simulink library "csc_hmg_homoraphy_meas_lib"  (R2015b)
settings: Solver=ode45  SolverMode=SingleTasking  StartTime=0.0  StopTime=10.0  RelTol=1e-3
values from neighbouring files (symbols this model uses):
  fsp_camera_alt_cutoff = 5    [csc_snp_sensor_prep_init.m]
  hmg_img1_delay_cnts = round(0.1 / est_time_step)    [csc_snp_sensor_prep_init.m]
  snp_fsp_index = [ 2 3 ]    [csc_snp_sensor_prep_init.m]
  snp_fsp_zero_index = [ 0 0 ]    [csc_snp_sensor_prep_init.m]
undefined symbols (not defined in the file or in its folder): cam_cam1_lander_dcm, cam_image_plane_norm, kfl_use_camera_meas
libraries: simulink x2, util_info_lib x2, csu_htv_homography_to_velocity_lib x2, csu_und_unduplicate_lib x2, util_common_lib x2
settings Model: ExtModeAutoUpdateStatusClock=off  Creator=Administrator  LastModifiedBy=Mark Agbayani
settings DataIOCC: SaveFormat=Array  SignalLoggingSaveFormat=ModelDataLogs
settings OptimizationCC: BlockReduction=off  BooleanDataType=off  ExpressionDepthLimit=2147483647
settings DebuggingCC: SaveWithParameterizedLinksMsg=none  UnderspecifiedInitializationDetection=Classic  MergeDetectMultiDrivingBlocksExec=none  SignalResolutionControl=TryResolveAllWithWarning  FcnCallInpInsideContextMsg=EnableAllAsWarning  StateNameClashWarn=warning  StrictBusMsg=Warning
settings HardwareCC: ProdBitPerPointer=32  ProdLargestAtomicFloat=None  ProdIntDivRoundTo=Undefined  ProdEndianess=Unspecified  ProdWordSize=32  ProdHWDeviceType=32-bit Generic  TargetUnknown=on
settings GRTTargetCC: GeneratePreprocessorConditionals=Disable all  CombineOutputUpdateFcns=off  GRTInterface=on
settings ConfigComp: CovModelRefEnable=Off  CovSFcnEnable=off

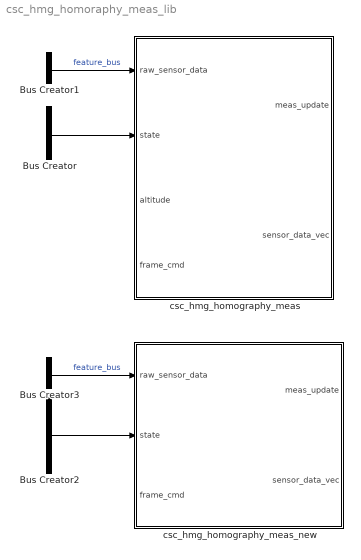
== system csc_hmg_homoraphy_meas_lib ==
  Bus Creator : BusCreator  Inputs=4
  Bus Creator1 : BusCreator  Inputs=2  OutDataTypeStr=Bus: feature_msg  NonVirtualBus=on
  Bus Creator2 : BusCreator  Inputs=5
  Bus Creator3 : BusCreator  Inputs=2  OutDataTypeStr=Bus: feature_msg  NonVirtualBus=on
  csc_hmg_homography_meas : Subsystem
  csc_hmg_homography_meas_new : Subsystem
  wires:
  ? -> Bus Creator/2  "accel"
  ? -> Bus Creator/3  "rate"
  ? -> Bus Creator/1  "x"
  ? -> Bus Creator/4  "q"
  Bus Creator/1 -> csc_hmg_homography_meas/2(state)
  ? -> Bus Creator1/2  "pixels_2"
  ? -> Bus Creator1/1  "pixels_1"
  Bus Creator1/1 -> csc_hmg_homography_meas/1(raw_sensor_data)  "feature_bus"
  ? -> Bus Creator2/2  "accel"
  ? -> Bus Creator2/3  "rate"
  ? -> Bus Creator2/1  "x"
  ? -> Bus Creator2/4  "q"
  Bus Creator2/1 -> csc_hmg_homography_meas_new/2(state)
  ? -> Bus Creator3/2  "pixels_2"
  ? -> Bus Creator3/1  "pixels_1"
  Bus Creator3/1 -> csc_hmg_homography_meas_new/1(raw_sensor_data)  "feature_bus"
  ? -> Bus Creator2/5  "altitude"

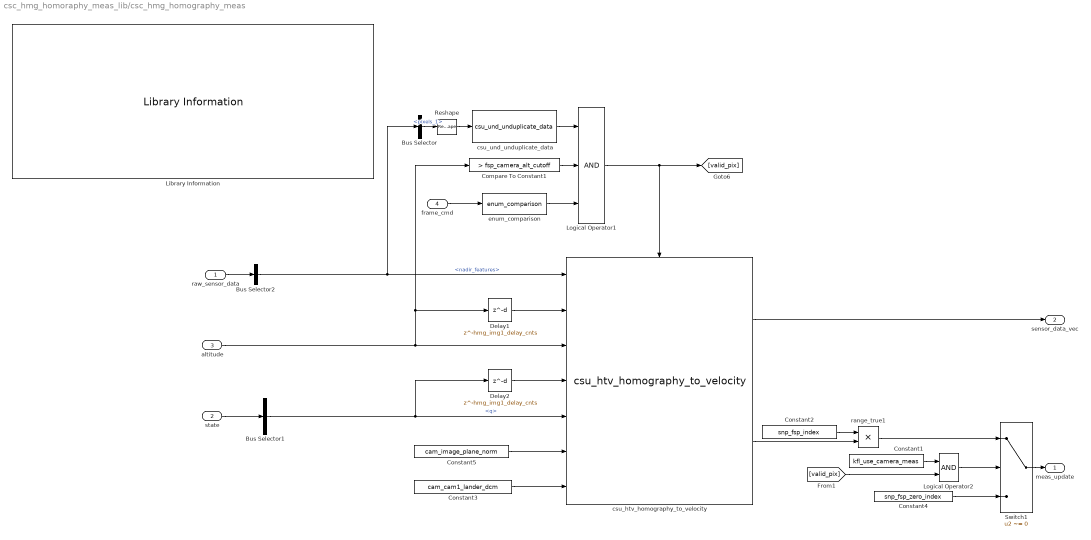
== system csc_hmg_homoraphy_meas_lib/csc_hmg_homography_meas ==
  raw_sensor_data : Inport
  state : Inport  Port=2
  altitude : Inport  Port=3
  frame_cmd : Inport  Port=4
  Bus Selector : BusSelector  OutputSignals=pixels_1
  Bus Selector1 : BusSelector  OutputSignals=q
  Bus Selector2 : BusSelector  OutputSignals=nadir_features
  Compare To Constant1 : simulink/Logic and Bit Operations/Compare To Constant  relop=>  const=fsp_camera_alt_cutoff  OutDataTypeStr=uint8
  Constant1 : Constant  Value=kfl_use_camera_meas
  Constant2 : Constant  Value=snp_fsp_index
  Constant3 : Constant  Value=cam_cam1_lander_dcm
  Constant4 : Constant  Value=snp_fsp_zero_index
  Constant5 : Constant  Value=cam_image_plane_norm  VectorParams1D=off
  Delay1 : Delay  DelayLength=hmg_img1_delay_cnts
  Delay2 : Delay  DelayLength=hmg_img1_delay_cnts
  Library Information : util_info_lib/Library Information  owner='NONE'
  Logical Operator1 : Logic  Inputs=3  AllPortsSameDT=off  OutDataTypeStr=boolean
  Logical Operator2 : Logic  AllPortsSameDT=off  OutDataTypeStr=boolean
  Reshape : Reshape
  Switch1 : Switch  Criteria=u2 ~= 0
  csu_htv_homography_to_velocity : csu_htv_homography_to_velocity_lib/csu_htv_homography_to_velocity
  csu_und_unduplicate_data : csu_und_unduplicate_lib/csu_und_unduplicate_data  initial_compare=0
  enum_comparison : util_common_lib/enum_comparison  comparison_type===
  range_true1 : Product  RndMeth=Zero
  meas_update : Outport
  sensor_data_vec : Outport  Port=2
  wires:
  [valid_pix] -> Logical Operator2/2
  Logical Operator2/1 -> Switch1/2
  Constant1/1 -> Logical Operator2/1
  Constant2/1 -> range_true1/1
  range_true1/1 -> Switch1/1
  csu_htv_homography_to_velocity/2 -> range_true1/2
  Delay2/1 -> csu_htv_homography_to_velocity/4
  frame_cmd/1 -> enum_comparison/1
  enum_comparison/1 -> Logical Operator1/3
  Constant3/1 -> csu_htv_homography_to_velocity/7
  Bus Selector2/1 -> csu_htv_homography_to_velocity/1, Bus Selector/1  "<nadir_features>"
  raw_sensor_data/1 -> Bus Selector2/1
  Constant5/1 -> csu_htv_homography_to_velocity/6
  Delay1/1 -> csu_htv_homography_to_velocity/2
  Bus Selector/1 -> Reshape/1  "<pixels_1>"
  Switch1/1 -> meas_update/1
  csu_htv_homography_to_velocity/1 -> sensor_data_vec/1
  Constant4/1 -> Switch1/3
  Compare To Constant1/1 -> Logical Operator1/2
  csu_und_unduplicate_data/1 -> Logical Operator1/1
  Logical Operator1/1 -> [valid_pix], csu_htv_homography_to_velocity/Enable
  Reshape/1 -> csu_und_unduplicate_data/1
  state/1 -> Bus Selector1/1
  Bus Selector1/1 -> csu_htv_homography_to_velocity/5, Delay2/1  "<q>"
  altitude/1 -> csu_htv_homography_to_velocity/3, Delay1/1, Compare To Constant1/1

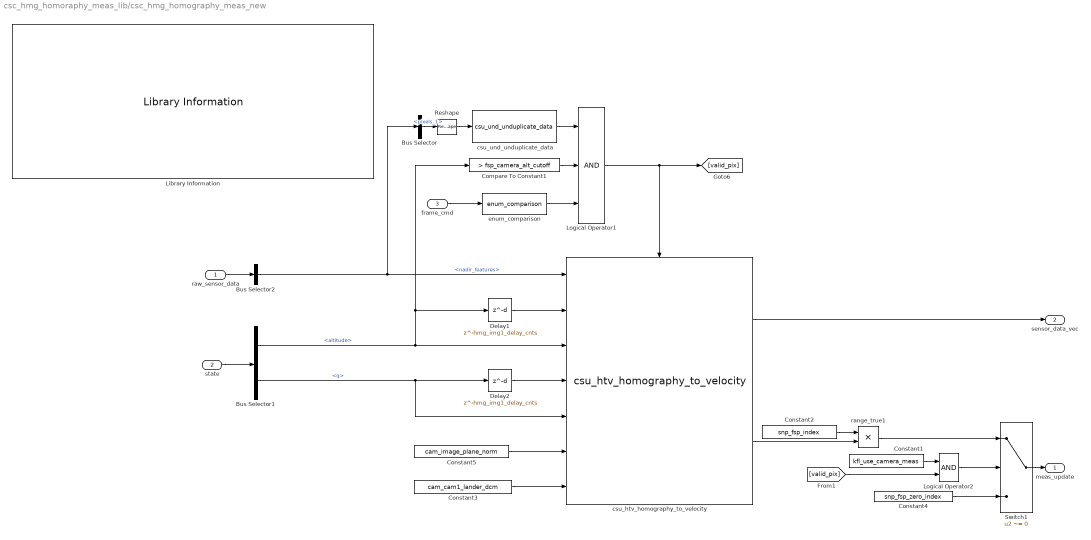
== system csc_hmg_homoraphy_meas_lib/csc_hmg_homography_meas_new ==
  raw_sensor_data : Inport
  state : Inport  Port=2
  frame_cmd : Inport  Port=3
  Bus Selector : BusSelector  OutputSignals=pixels_1
  Bus Selector1 : BusSelector  OutputSignals=altitude,q
  Bus Selector2 : BusSelector  OutputSignals=nadir_features
  Compare To Constant1 : simulink/Logic and Bit Operations/Compare To Constant  relop=>  const=fsp_camera_alt_cutoff  OutDataTypeStr=uint8
  Constant1 : Constant  Value=kfl_use_camera_meas
  Constant2 : Constant  Value=snp_fsp_index
  Constant3 : Constant  Value=cam_cam1_lander_dcm
  Constant4 : Constant  Value=snp_fsp_zero_index
  Constant5 : Constant  Value=cam_image_plane_norm  VectorParams1D=off
  Delay1 : Delay  DelayLength=hmg_img1_delay_cnts
  Delay2 : Delay  DelayLength=hmg_img1_delay_cnts
  Library Information : util_info_lib/Library Information  owner='NONE'
  Logical Operator1 : Logic  Inputs=3  AllPortsSameDT=off  OutDataTypeStr=boolean
  Logical Operator2 : Logic  AllPortsSameDT=off  OutDataTypeStr=boolean
  Reshape : Reshape
  Switch1 : Switch  Criteria=u2 ~= 0
  csu_htv_homography_to_velocity : csu_htv_homography_to_velocity_lib/csu_htv_homography_to_velocity
  csu_und_unduplicate_data : csu_und_unduplicate_lib/csu_und_unduplicate_data  initial_compare=0
  enum_comparison : util_common_lib/enum_comparison  comparison_type===
  range_true1 : Product  RndMeth=Zero
  meas_update : Outport
  sensor_data_vec : Outport  Port=2
  wires:
  [valid_pix] -> Logical Operator2/2
  Logical Operator2/1 -> Switch1/2
  Constant1/1 -> Logical Operator2/1
  Constant2/1 -> range_true1/1
  range_true1/1 -> Switch1/1
  csu_htv_homography_to_velocity/2 -> range_true1/2
  Delay2/1 -> csu_htv_homography_to_velocity/4
  frame_cmd/1 -> enum_comparison/1
  enum_comparison/1 -> Logical Operator1/3
  Constant3/1 -> csu_htv_homography_to_velocity/7
  Bus Selector2/1 -> csu_htv_homography_to_velocity/1, Bus Selector/1  "<nadir_features>"
  raw_sensor_data/1 -> Bus Selector2/1
  Constant5/1 -> csu_htv_homography_to_velocity/6
  Delay1/1 -> csu_htv_homography_to_velocity/2
  Bus Selector/1 -> Reshape/1  "<pixels_1>"
  Switch1/1 -> meas_update/1
  csu_htv_homography_to_velocity/1 -> sensor_data_vec/1
  Constant4/1 -> Switch1/3
  Compare To Constant1/1 -> Logical Operator1/2
  csu_und_unduplicate_data/1 -> Logical Operator1/1
  Logical Operator1/1 -> [valid_pix], csu_htv_homography_to_velocity/Enable
  Reshape/1 -> csu_und_unduplicate_data/1
  state/1 -> Bus Selector1/1
  Bus Selector1/2 -> Delay2/1, csu_htv_homography_to_velocity/5  "<q>"
  Bus Selector1/1 -> csu_htv_homography_to_velocity/3, Delay1/1, Compare To Constant1/1  "<altitude>"
